simulink model "refulinear"  (Simulink 2.20)
settings: Solver=ode45  StartTime=0.0  StopTime=10  RelTol=1e-3  AbsTol=1e-6
values from neighbouring files (symbols this model uses):
  kdc = dcgain(clsystem)    [leadreg.m]    (also in reference.m)
undefined symbols (not defined in the file or in its folder): denr, numr
libraries: simulink_extras x3
settings Model: ConsistencyChecking=off  RTWPlaceOutputsASAP=off

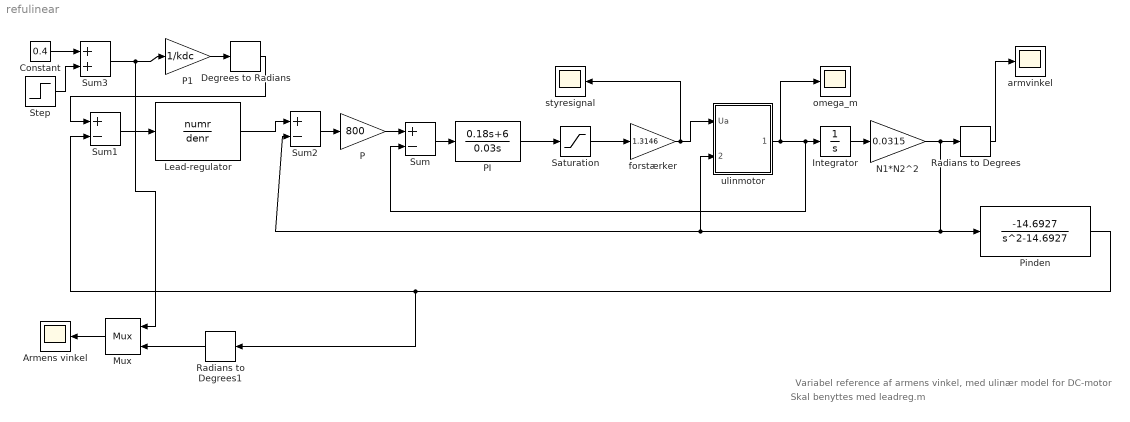
== system refulinear ==
  note: Variabel reference af armens vinkel, med ulinær model for DC-motor
  note: Skal benyttes med leadreg.m
  Armens vinkel : Scope
      settings: TickLabels=on  TimeRange=5  YMin=-1  YMax=1  SaveToWorkspace=off  SaveName=ScopeData
  Constant : Constant  Value=0.4
  Degrees to Radians : simulink_extras/Transformations/Degrees to Radians
  Integrator : Integrator  ExternalReset=none  InitialConditionSource=internal  InitialCondition=0  LimitOutput=off  UpperSaturationLimit=inf  LowerSaturationLimit=-inf  ShowSaturationPort=off  ShowStatePort=off  AbsoluteTolerance=auto
  Lead-regulator : TransferFcn  Numerator=numr  Denominator=denr
  Mux : Mux  Orientation=left  Inputs=2
  N1*N2^2 : Gain  Gain=0.0315
  P : Gain  Gain=800
  P1 : Gain  Gain=1/kdc
  PI : TransferFcn  Numerator=[0.18 6]  Denominator=[0.03 0]
  Pinden : TransferFcn  Numerator=[-14.6927]  Denominator=[1 0 -14.6927 ]
  Radians to Degrees : simulink_extras/Transformations/Radians to Degrees
  Radians to Degrees1 : simulink_extras/Transformations/Radians to Degrees  Orientation=left
  Saturation : Saturate  UpperLimit=5  LowerLimit=-5
  Step : Step  Time=5  Before=0  After=-0.7
  Sum : Sum  Inputs=+-
  Sum1 : Sum  Inputs=+-
  Sum2 : Sum  Inputs=+-
  Sum3 : Sum  Inputs=++
  armvinkel : Scope
      settings: TickLabels=on  TimeRange=10  YMin=-0.00065  YMax=0  SaveToWorkspace=off  SaveName=ScopeData
  forstærker : Gain  Gain=1.3146
  "omega_m " : Scope
      settings: TickLabels=on  TimeRange=10  YMin=-0.00065  YMax=0  SaveToWorkspace=off  SaveName=ScopeData
  styresignal : Scope
      settings: TickLabels=on  TimeRange=0.5  YMin=0  YMax=13  SaveToWorkspace=off  SaveName=ScopeData
  ulinmotor : Subsystem
  wires:
  Sum/1 -> PI/1
  Saturation/1 -> forstærker/1
  forstærker/1 -> styresignal/1, ulinmotor/1(Ua)
  Integrator/1 -> N1*N2^2/1
  Radians to Degrees/1 -> armvinkel/1
  PI/1 -> Saturation/1
  N1*N2^2/1 -> Radians to Degrees/1, Pinden/1, Sum2/2, ulinmotor/2(Theta_a)
  ulinmotor/1(Omega) -> "omega_m "/1, Integrator/1, Sum/2
  P/1 -> Sum/1
  Sum2/1 -> P/1
  Degrees to Radians/1 -> Sum1/1
  Lead-regulator/1 -> Sum2/1
  Pinden/1 -> Sum1/2, Radians to Degrees1/1
  Sum1/1 -> Lead-regulator/1
  P1/1 -> Degrees to Radians/1
  Step/1 -> Sum3/2
  Constant/1 -> Sum3/1
  Sum3/1 -> P1/1, Mux/1
  Radians to Degrees1/1 -> Mux/2
  Mux/1 -> Armens vinkel/1

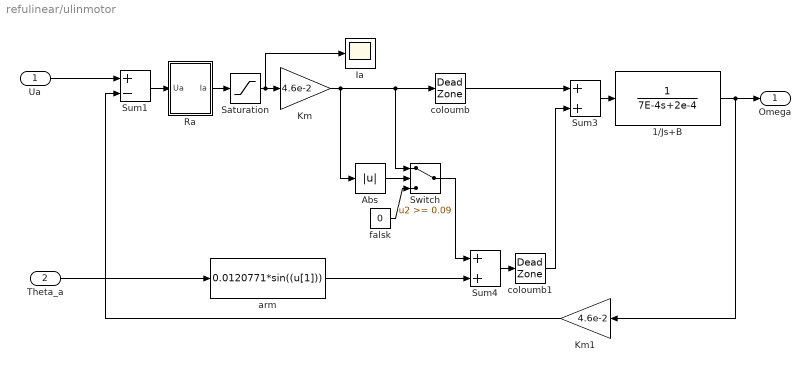
== system refulinear/ulinmotor ==
  Ua : Inport  Port=1  PortWidth=-1  SampleTime=-1
  Theta_a : Inport  Port=2  PortWidth=-1  SampleTime=-1
  1/Js+B : TransferFcn  Numerator=[1]  Denominator=[7E-4 2e-4]
  Abs : Abs
  Ia : Scope
      settings: TickLabels=on  TimeRange=5  YMin=-3  YMax=3  SaveToWorkspace=off  SaveName=ScopeData
  Km : Gain  Gain=4.6e-2
  Km1 : Gain  Orientation=left  Gain=4.6e-2
  Ra : Subsystem
  Saturation : Saturate  UpperLimit=6.5  LowerLimit=-6.5
  Sum1 : Sum  Inputs=+-
  Sum3 : Sum  Inputs=++
  Sum4 : Sum  Inputs=++
  Switch : Switch  Threshold=0.09
  arm : Fcn  Expr=0.0120771*sin((u[1]))
  coloumb : DeadZone  LowerValue=-0.09  UpperValue=0.09
  coloumb1 : DeadZone  LowerValue=-2.857  UpperValue=2.857
  falsk : Constant  Value=0
  Omega : Outport  Port=1  InitialOutput=0
  wires:
  Sum3/1 -> 1/Js+B/1
  Ua/1 -> Sum1/1
  Sum1/1 -> Ra/1(Ua)
  Theta_a/1 -> arm/1
  1/Js+B/1 -> Omega/1, Km1/1
  coloumb/1 -> Sum3/1
  coloumb1/1 -> Sum3/2
  arm/1 -> Sum4/2
  Sum4/1 -> coloumb1/1
  Km/1 -> Abs/1, coloumb/1, Switch/1
  Abs/1 -> Switch/2
  falsk/1 -> Switch/3
  Switch/1 -> Sum4/1
  Ra/1(Ia) -> Saturation/1
  Saturation/1 -> Km/1, Ia/1
  Km1/1 -> Sum1/2

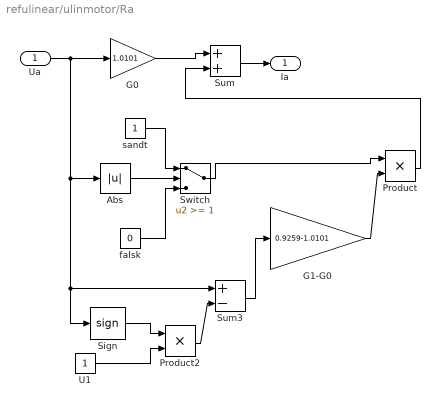
== system refulinear/ulinmotor/Ra ==
  Ua : Inport  Port=1  PortWidth=-1  SampleTime=-1
  Abs : Abs
  G0 : Gain  Gain=1.0101
  G1-G0 : Gain  Gain=0.9259-1.0101
  Product : Product  Inputs=2
  Product2 : Product  Inputs=2
  Sign : Signum
  Sum : Sum  Inputs=++
  Sum3 : Sum  Inputs=+-
  Switch : Switch  Threshold=1
  U1 : Constant  Value=1
  falsk : Constant  Value=0
  sandt : Constant  Value=1
  Ia : Outport  Port=1  InitialOutput=0
  wires:
  Product/1 -> Sum/2
  G1-G0/1 -> Product/2
  Sum3/1 -> G1-G0/1
  Product2/1 -> Sum3/2
  U1/1 -> Product2/2
  Sign/1 -> Product2/1
  Switch/1 -> Product/1
  sandt/1 -> Switch/1
  falsk/1 -> Switch/3
  Abs/1 -> Switch/2
  Ua/1 -> Sign/1, Sum3/1, Abs/1, G0/1
  G0/1 -> Sum/1
  Sum/1 -> Ia/1
